simulink model "IEEE24bus_simplified"  (R2019b)
settings: Solver=ode23tb  StartTime=0.0  StopTime=100  MaxStep=1/60  RelTol=1e-4  AbsTol=1e-3  EnableMultiTasking=on
PreLoadFcn:
  | RTS96_data
values from neighbouring files (symbols this model uses):
  Efmax = 5    [IEEE24_bus.m]    (also in IEEE24bus_simplified_benchmark.m)
  Efmin = -5    [IEEE24_bus.m]    (also in IEEE24bus_simplified_benchmark.m)
  EXc_sys = [     0.06  25  0.2    0.0505  0.5685   0 0   0.091  0.35 ... (first row only)    [IEEE24bus_simplified_benchmark.m]
  FH1 = 12    [IEEE24bus_simplified_benchmark.m]
  FI1 = .9    (= 0.9)    [IEEE24bus_simplified_benchmark.m]
  FL1 = .1    (= 0.1)    [IEEE24bus_simplified_benchmark.m]
  KH1 = 100    [IEEE24bus_simplified_benchmark.m]
  KI1 = 1    [IEEE24_bus.m]    (also in IEEE24bus_simplified_benchmark.m = 20)
  KL1 = 10    [IEEE24bus_simplified_benchmark.m]
undefined symbols (not defined in the file or in its folder): D1, Delta
libraries: powerlib x157, sps_avr x11, powerlib_extras x1
(part 3 of 3)

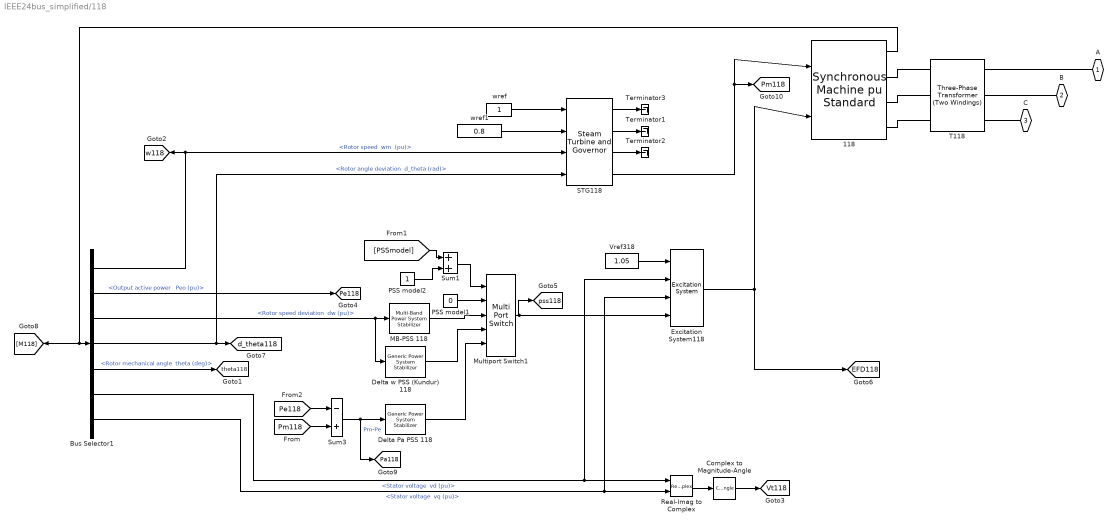
== system IEEE24bus_simplified/118 ==
  118 : powerlib/Machines/Synchronous Machine pu Standard  PresetModel=No  MechanicalLoad=Mechanical power Pm  ShowDetailedParameters=on  RotorType=Round  Units=per unit standard parameters  MeasurementBus=off  NominalParameters="[ 500E6  18e3   60]"  Reactances1="[ 1.782, 0.444, 0.283, 1.739, 1.201, 0.277,  0.275 ]"  Reactances2="[ 1.782, 0.444, 0.283, 1.739,  0.277,  0.275 ]"  dAxisTimeConstants=Open-circuit  qAxisTimeConstants=Open-circuit  TimeConstants1="[  6.070  0.055  0.035  ]"  TimeConstants2="[  6.070  0.055  1.5    0.152  ]"  TimeConstants3="[  6.070  0.055  0.035  ]"  TimeConstants4=[ 8.0, 0.03, 0.3371, 0.0295 ]  TimeConstants5=[ 1.01, 0.053, 0.1 ]  TimeConstants6=[ 1.3201, 0.023, 1.0, 0.07 ]  TimeConstants7="[  1.01  0.053  0.051266  ]"  TimeConstants8=[ 1.3201, 0.0231, 0.3371, 0.0295 ]  StatorResistance=0.0041  Mechanical="[ 1990/(500) 0  4 ]"  PolePairs=4  InitialConditions=[0 -39.3029 0.797786 0.797786 0.797786 -8.667 -128.667 111.333 2.00378]  SetSaturation=off  Saturation=[0.6404,0.7127,0.8441,0.9214,0.9956,1.082,1.19,1.316,1.457;0.7,0.7698,0.8872,0.9466,0.9969,1.046,1.1,1.151,1.201]  LoadFlowParameters=[1 400000000 18900 0 0]  TsPowergui=0  TsBlock=-1  IterativeModel=Forward Euler  IterativeDiscreteModel=Trapezoidal non iterative  BusType=PV  Pref=400E6  Qref=0  Qmin=-50e6  Qmax=200E6  PLF=0  QLF=0
      settings: SourceProductName=Simscape Electrical
  Bus Selector1 : BusSelector  OutputSignals="Mechanical.Rotor speed  wm  (pu),Output active power   Peo (pu),Mechanical.Rotor speed deviation  dw (pu),Mechanical.Rotor angle deviation  d_theta (rad),Mechanical.Rotor mechanical angle  theta (deg),dq0 components.Stator voltage  vd (pu),dq0 components.Stator voltage  vq (pu)"
  Complex to Magnitude-Angle : ComplexToMagnitudeAngle  Output=Magnitude
  Delta Pa PSS 118 : powerlib/Machines/Generic Power System Stabilizer  Tsensor=15e-3  K=2.5*1.25  Twashout=1  Tleadlag1=[60e-3 1]  Tleadlag2=[0 0]  VSlimits=[-0.15 0.15]  Vinit=0  Plot_On=off  MagdB_On=on  FreqRange=logspace(-2,2,500)
      settings: SourceProductName=Simscape Electrical  SourceProductBaseCode=PS
  Delta w PSS (Kundur) 118 : powerlib/Machines/Generic Power System Stabilizer  Tsensor=15e-3  K=30  Twashout=10  Tleadlag1=[50e-3 20e-3]  Tleadlag2=[3 5.4]  VSlimits=[-0.15 0.15]  Vinit=0  Plot_On=off  MagdB_On=on  FreqRange=logspace(-2,2,500)
      settings: SourceProductName=Simscape Electrical  SourceProductBaseCode=PS
  Excitation System118 : sps_avr/Excitation System  tr=EXc_sys(8,1)  reg="[ EXc_sys(8,2)   EXc_sys(8,3) ]"  exc="[ EXc_sys(8,4)  EXc_sys(8,5)]"  tgr="[ EXc_sys(8,6)  EXc_sys(8,7) ]"  damp="[ EXc_sys(8,8)   EXc_sys(8,9)]"  sat=[ 0, 0 ]  lim="[ Efmin Efmax   0 ]"  v0=[1.05,2.00378]
      settings: SourceProductName=Simscape Electrical  SourceProductBaseCode=PS
  MB-PSS 118 : powerlib/Machines/Multi-Band Power System Stabilizer  OperationMode=Simplified settings  Kg=G1  GL=[FL1 KL1]  GI=[FI1 KI1]  GH=[FH1 KH1]  GLd=[66 66 9.4]  TcLF=[1.667 2 0 0 0 0 2 2.4 0 0 0 0 1 1]  GId=[66 66 47.6]  TcIF=[1 1 0.25 0.3 0 0 1 1 0.3 0.36 0 0 0 0]  GHd=[66 66 233]  TcHF="[0.01 0.012 0 0 0 0  0.012 0.0144 0 0 0 0 1 1]"  LIM=[.075 .15 .15 .15]  Plot_On=off  MagdB_On=off  FreqRange=logspace(-2,2,500)
      settings: SourceProductName=Simscape Electrical  SourceProductBaseCode=PS
  Multiport Switch1 : MultiPortSwitch  Inputs=4  InputSameDT=on
  PSS model1 : Constant  Value=0
  PSS model2 : Constant
  Real-Imag to Complex : RealImagToComplex
  STG118 : powerlib/Machines/Steam Turbine and Governor  gentype=Tandem-compound (single mass)  reg1="[ 1  0.05    0 ]"  reg2="[ 0.001  0.15 ]"  reg3="[ -0.1  0.1  0  4.496 ]"  N=3600  turb1="[ 0  10   3.3   0.5   ]"  turb2="[   0   0.36    0.36   0.28   ]"  HA="[ 0.046  1.430  1.465   0.192 ]"  KA="[ 90.44  53.88  64.59   62.94  ]"  DA="[ 0.0115  0.3575  0.3663   0.0137  ]"  ini1=0.802609  ini2=[0.779316,-31.4247]
      settings: SourceProductName=Simscape Electrical  SourceProductBaseCode=PS
  Sum1 : Sum  SaturateOnIntegerOverflow=on  InputSameDT=on  OutDataTypeStr=Inherit: Same as first input
  Sum3 : Sum  Inputs=-+  SaturateOnIntegerOverflow=on  InputSameDT=on  OutDataTypeStr=Inherit: Same as first input
  T118 : powerlib/Elements/Three-Phase Transformer (Two Windings)  Winding1Connection=Delta (D1)  Winding2Connection=Yg  CoreType=Three single-phase transformers  SetSaturation=off  Hysteresis=off  DataFile='hysteresis'  SetInitialFlux=off  Measurements=None  UNITS=pu  NominalPower=[ 471E6 , 60 ]  Winding1=[ 18e3 , 1e-6 , 0 ]  Winding2=[ 230e3 , 0, 0.15 ]  Rm=500  Lm=500  L0=0.5  Saturation=[ 0,0 ; 0.0024,1.2 ; 1.0,1.52 ]  InitialFluxes=[ 0.8 , -0.8 , 0.7 ]  BreakLoop=off  DiscreteSolver=Trapezoidal iterative  DataType=off  TransfoNumber=0
      settings: SourceProductName=Simscape Electrical
  Terminator1 : Terminator
  Terminator2 : Terminator
  Terminator3 : Terminator
  Vref318 : Constant  Value=1.05
  wref : Constant
  wref1 : Constant  Value=0.8
  A : PMIOPort  Side=Right
  B : PMIOPort  Port=2  Side=Right
  C : PMIOPort  Port=3  Side=Right
  tag scope: EFD118=global, Pa118=global, Pe118=global, Pm118=global, Vt118=global, d_theta118=global, pss118=global, theta118=global, w118=global
  wires:
  Vref318/1 -> Excitation System118/1
  wref1/1 -> STG118/2
  wref/1 -> STG118/1
  118/1 -> [M118], Bus Selector1/1
  Bus Selector1/1 -> STG118/3, [w118]  "<Rotor speed  wm  (pu)>"
  Bus Selector1/2 -> [Pe118]  "<Output active power   Peo (pu)>"
  Bus Selector1/3 -> Delta w PSS (Kundur) 118/1, MB-PSS 118/1  "<Rotor speed deviation  dw (pu)>"
  Multiport Switch1/1 -> [pss118], Excitation System118/4
  PSS model2/1 -> Sum1/2
  Sum1/1 -> Multiport Switch1/1
  [PSSmodel] -> Sum1/1
  PSS model1/1 -> Multiport Switch1/2
  MB-PSS 118/1 -> Multiport Switch1/3
  Bus Selector1/4 -> [d_theta118], STG118/4  "<Rotor angle deviation  d_theta (rad)>"
  Bus Selector1/5 -> [theta118]  "<Rotor mechanical angle  theta (deg)>"
  Real-Imag to Complex/1 -> Complex to Magnitude-Angle/1
  Complex to Magnitude-Angle/1 -> [Vt118]
  Bus Selector1/6 -> Excitation System118/2, Real-Imag to Complex/1  "<Stator voltage  vd (pu)>"
  Bus Selector1/7 -> Excitation System118/3, Real-Imag to Complex/2  "<Stator voltage  vq (pu)>"
  Excitation System118/1 -> 118/2, [EFD118]
  STG118/1 -> Terminator3/1
  STG118/2 -> Terminator1/1
  STG118/3 -> Terminator2/1
  Sum3/1 -> [Pa118], Delta Pa PSS 118/1  "Pm-Pe"
  Delta Pa PSS 118/1 -> Multiport Switch1/5
  Delta w PSS (Kundur) 118/1 -> Multiport Switch1/4
  STG118/4 -> 118/1, [Pm118]
  [Pm118] -> Sum3/2
  [Pe118] -> Sum3/1
  connections:
  118/RConn3 -- T118/LConn3
  B/RConn1 -- T118/RConn2
  118/RConn2 -- T118/LConn2
  118/RConn1 -- T118/LConn1
  A/RConn1 -- T118/RConn1
  C/RConn1 -- T118/RConn3

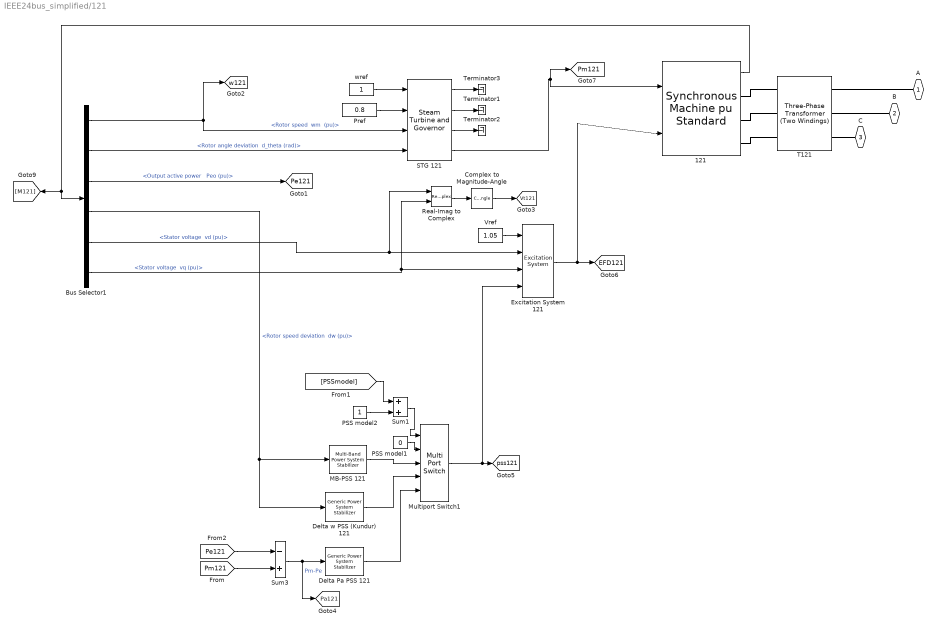
== system IEEE24bus_simplified/121 ==
  121 : powerlib/Machines/Synchronous Machine pu Standard  PresetModel=No  MechanicalLoad=Mechanical power Pm  ShowDetailedParameters=on  RotorType=Round  Units=per unit standard parameters  MeasurementBus=off  NominalParameters="[ 500E6  18e3   60]"  Reactances1="[ 1.782, 0.444, 0.283, 1.739, 1.201, 0.277,  0.275 ]"  Reactances2="[ 1.782, 0.444, 0.283, 1.739,  0.277,  0.275 ]"  dAxisTimeConstants=Open-circuit  qAxisTimeConstants=Open-circuit  TimeConstants1="[  6.070  0.055  0.035  ]"  TimeConstants2="[  6.070  0.055  1.5    0.152  ]"  TimeConstants3="[  6.070  0.055  0.035  ]"  TimeConstants4=[ 8.0, 0.03, 0.3371, 0.0295 ]  TimeConstants5=[ 1.01, 0.053, 0.1 ]  TimeConstants6=[ 1.3201, 0.023, 1.0, 0.07 ]  TimeConstants7="[  1.01  0.053  0.051266  ]"  TimeConstants8=[ 1.3201, 0.0231, 0.3371, 0.0295 ]  StatorResistance=0.0041  Mechanical="[ 1990/(500) 0  4 ]"  PolePairs=4  InitialConditions=[0 -38.0053 0.791351 0.791351 0.791351 -6.58132 -126.581 113.419 1.97426]  SetSaturation=off  Saturation=[0.6404,0.7127,0.8441,0.9214,0.9956,1.082,1.19,1.316,1.457;0.7,0.7698,0.8872,0.9466,0.9969,1.046,1.1,1.151,1.201]  LoadFlowParameters=[1 400000000 18900 0 0]  TsPowergui=0  TsBlock=-1  IterativeModel=Forward Euler  IterativeDiscreteModel=Trapezoidal non iterative  BusType=PV  Pref=400E6  Qref=0  Qmin=-50E6  Qmax=200E6  PLF=0  QLF=0
      settings: SourceProductName=Simscape Electrical
  Bus Selector1 : BusSelector  OutputSignals="Mechanical.Rotor speed  wm  (pu),Mechanical.Rotor angle deviation  d_theta (rad),Output active power   Peo (pu),Mechanical.Rotor speed deviation  dw (pu),dq0 components.Stator voltage  vd (pu),dq0 components.Stator voltage  vq (pu)"
  Complex to Magnitude-Angle : ComplexToMagnitudeAngle  Output=Magnitude
  Delta Pa PSS 121 : powerlib/Machines/Generic Power System Stabilizer  Tsensor=15e-3  K=2.5*1.25  Twashout=1  Tleadlag1=[60e-3 1]  Tleadlag2=[0 0]  VSlimits=[-0.15 0.15]  Vinit=0  Plot_On=off  MagdB_On=on  FreqRange=logspace(-2,2,500)
      settings: SourceProductName=Simscape Electrical  SourceProductBaseCode=PS
  Delta w PSS (Kundur) 121 : powerlib/Machines/Generic Power System Stabilizer  Tsensor=15e-3  K=30  Twashout=10  Tleadlag1=[50e-3 20e-3]  Tleadlag2=[3 5.4]  VSlimits=[-0.15 0.15]  Vinit=0  Plot_On=off  MagdB_On=on  FreqRange=logspace(-2,2,500)
      settings: SourceProductName=Simscape Electrical  SourceProductBaseCode=PS
  Excitation System 121 : sps_avr/Excitation System  tr=EXc_sys(9,1)  reg="[ EXc_sys(9,2)   EXc_sys(9,3) ]"  exc="[ EXc_sys(9,4)  EXc_sys(9,5)]"  tgr="[ EXc_sys(9,6)  EXc_sys(9,7) ]"  damp="[ EXc_sys(9,8)   EXc_sys(9,9)]"  sat=[ 0, 0 ]  lim="[ Efmin Efmax   0 ]"  v0=[1.05,1.97426]
      settings: SourceProductName=Simscape Electrical  SourceProductBaseCode=PS
  MB-PSS 121 : powerlib/Machines/Multi-Band Power System Stabilizer  OperationMode=Simplified settings  Kg=G1  GL=[FL1 KL1]  GI=[FI1 KI1]  GH=[FH1 KH1]  GLd=[66 66 9.4]  TcLF=[1.667 2 0 0 0 0 2 2.4 0 0 0 0 1 1]  GId=[66 66 47.6]  TcIF=[1 1 0.25 0.3 0 0 1 1 0.3 0.36 0 0 0 0]  GHd=[66 66 233]  TcHF="[0.01 0.012 0 0 0 0  0.012 0.0144 0 0 0 0 1 1]"  LIM=[.075 .15 .15 .15]  Plot_On=off  MagdB_On=off  FreqRange=logspace(-2,2,500)
      settings: SourceProductName=Simscape Electrical  SourceProductBaseCode=PS
  Multiport Switch1 : MultiPortSwitch  Inputs=4  InputSameDT=on
  PSS model1 : Constant  Value=0
  PSS model2 : Constant
  Pref : Constant  Value=0.8
  Real-Imag to Complex : RealImagToComplex
  STG 121 : powerlib/Machines/Steam Turbine and Governor  gentype=Tandem-compound (single mass)  reg1="[ 1  0.05    0 ]"  reg2="[ 0.001  0.15 ]"  reg3="[ -0.1  0.1  0  4.496 ]"  N=3600  turb1="[ 0  10   3.3   0.5   ]"  turb2="[   0   0.36    0.36   0.28   ]"  HA="[ 0.046  1.430  1.465   0.192 ]"  KA="[ 90.44  53.88  64.59   62.94  ]"  DA="[ 0.0115  0.3575  0.3663   0.0137  ]"  ini1=0.802568  ini2=[0.779316,-31.4247]
      settings: SourceProductName=Simscape Electrical  SourceProductBaseCode=PS
  Sum1 : Sum  SaturateOnIntegerOverflow=on  InputSameDT=on  OutDataTypeStr=Inherit: Same as first input
  Sum3 : Sum  Inputs=-+  SaturateOnIntegerOverflow=on  InputSameDT=on  OutDataTypeStr=Inherit: Same as first input
  T121 : powerlib/Elements/Three-Phase Transformer (Two Windings)  Winding1Connection=Delta (D1)  Winding2Connection=Yg  CoreType=Three single-phase transformers  SetSaturation=off  Hysteresis=off  DataFile='hysteresis'  SetInitialFlux=off  Measurements=None  UNITS=pu  NominalPower="[ 471E6  , 60 ]"  Winding1=[ 18e3 , 1e-6 , 0 ]  Winding2=[ 230e3 , 0, 0.15 ]  Rm=500  Lm=500  L0=0.5  Saturation=[ 0,0 ; 0.0024,1.2 ; 1.0,1.52 ]  InitialFluxes=[ 0.8 , -0.8 , 0.7 ]  BreakLoop=off  DiscreteSolver=Trapezoidal iterative  DataType=off  TransfoNumber=0
      settings: SourceProductName=Simscape Electrical
  Terminator1 : Terminator
  Terminator2 : Terminator
  Terminator3 : Terminator
  Vref : Constant  Value=1.05
  wref : Constant
  A : PMIOPort  Side=Right
  B : PMIOPort  Port=2  Side=Right
  C : PMIOPort  Port=3  Side=Right
  tag scope: EFD121=global, Pa121=global, Pe121=global, Pm121=global, Vt121=global, pss121=global, w121=global
  wires:
  Excitation System 121/1 -> 121/2, [EFD121]
  Vref/1 -> Excitation System 121/1
  STG 121/2 -> Terminator1/1
  STG 121/3 -> Terminator2/1
  STG 121/1 -> Terminator3/1
  wref/1 -> STG 121/1
  Pref/1 -> STG 121/2
  121/1 -> [M121], Bus Selector1/1
  Bus Selector1/1 -> STG 121/3, [w121]  "<Rotor speed  wm  (pu)>"
  Bus Selector1/2 -> STG 121/4  "<Rotor angle deviation  d_theta (rad)>"
  PSS model2/1 -> Sum1/2
  Sum1/1 -> Multiport Switch1/1
  Multiport Switch1/1 -> Excitation System 121/4, [pss121]
  [PSSmodel] -> Sum1/1
  PSS model1/1 -> Multiport Switch1/2
  MB-PSS 121/1 -> Multiport Switch1/3
  Bus Selector1/5 -> Real-Imag to Complex/1, Excitation System 121/2  "<Stator voltage  vd (pu)>"
  Bus Selector1/6 -> Real-Imag to Complex/2, Excitation System 121/3  "<Stator voltage  vq (pu)>"
  Real-Imag to Complex/1 -> Complex to Magnitude-Angle/1
  Complex to Magnitude-Angle/1 -> [Vt121]
  Bus Selector1/3 -> [Pe121]  "<Output active power   Peo (pu)>"
  Bus Selector1/4 -> Delta w PSS (Kundur) 121/1, MB-PSS 121/1  "<Rotor speed deviation  dw (pu)>"
  Sum3/1 -> [Pa121], Delta Pa PSS 121/1  "Pm-Pe"
  Delta Pa PSS 121/1 -> Multiport Switch1/5
  Delta w PSS (Kundur) 121/1 -> Multiport Switch1/4
  STG 121/4 -> [Pm121], 121/1
  [Pm121] -> Sum3/2
  [Pe121] -> Sum3/1
  connections:
  121/RConn3 -- T121/LConn3
  T121/RConn1 -- A/RConn1
  121/RConn2 -- T121/LConn2
  121/RConn1 -- T121/LConn1
  T121/RConn2 -- B/RConn1
  T121/RConn3 -- C/RConn1

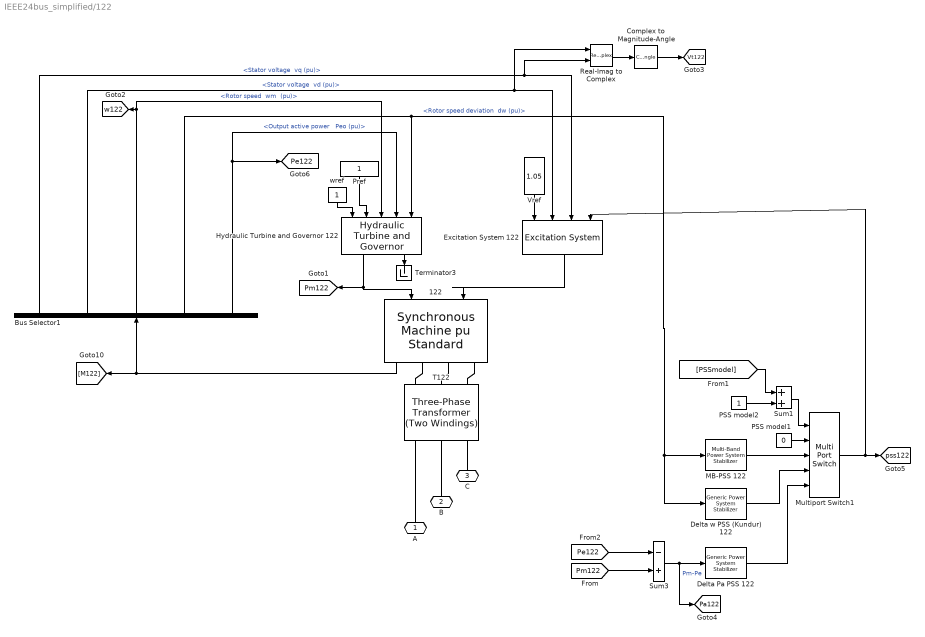
== system IEEE24bus_simplified/122 ==
  122 : powerlib/Machines/Synchronous Machine pu Standard  PresetModel=No  MechanicalLoad=Mechanical power Pm  ShowDetailedParameters=on  RotorType=Salient-pole  Units=per unit standard parameters  MeasurementBus=off  NominalParameters="[ 300E6  18e3   60]"  Reactances1="[ 0.995, 0.195, 0.155, 0.568,  0.568,  0.143,  0.160 ]"  Reactances2="[ 0.995, 0.195, 0.155, 0.568,  0.143,  0.160 ]"  dAxisTimeConstants=Open-circuit  qAxisTimeConstants=Open-circuit  TimeConstants1="[  9.2  0.03  0.06  ]"  TimeConstants2="[9.2     0.03    2       0.06]"  TimeConstants3="[  9.2  0.01  0.01  ]"  TimeConstants4="[  9.2  0.03  0.06  1 ]"  TimeConstants5=[ 1.01, 0.053, 0.1 ]  TimeConstants6=[ 1.3201, 0.023, 1.0, 0.07 ]  TimeConstants7="[  1.01  0.053  0.051266  ]"  TimeConstants8=[ 1.3201, 0.0231, 0.3371, 0.0295 ]  StatorResistance=0.0014  Mechanical="[ 1603/250 0  20]"  PolePairs=20  InitialConditions=[0 -51.0485 0.960961 0.960961 0.960961 5.59863 -114.401 125.599 1.47302]  SetSaturation=off  Saturation=[0.6404,0.7127,0.8441,0.9214,0.9956,1.082,1.19,1.316,1.457;0.7,0.7698,0.8872,0.9466,0.9969,1.046,1.1,1.151,1.201]  LoadFlowParameters=[1 300000000 18900 0 0]  TsPowergui=0  TsBlock=-1  IterativeModel=Forward Euler  IterativeDiscreteModel=Trapezoidal non iterative  BusType=PV  Pref=300E6  Qref=0  Qmin=-60E6  Qmax=96E6  PLF=0  QLF=0
      settings: SourceProductName=Simscape Electrical
  Bus Selector1 : BusSelector  OutputSignals="dq0 components.Stator voltage  vq (pu),dq0 components.Stator voltage  vd (pu),Mechanical.Rotor speed  wm  (pu),Mechanical.Rotor speed deviation  dw (pu),Output active power   Peo (pu)"
  Complex to Magnitude-Angle : ComplexToMagnitudeAngle  Output=Magnitude
  Delta Pa PSS 122 : powerlib/Machines/Generic Power System Stabilizer  Tsensor=15e-3  K=2.5*1.25  Twashout=1  Tleadlag1=[60e-3 1]  Tleadlag2=[0 0]  VSlimits=[-0.15 0.15]  Vinit=0  Plot_On=off  MagdB_On=on  FreqRange=logspace(-2,2,500)
      settings: SourceProductName=Simscape Electrical  SourceProductBaseCode=PS
  Delta w PSS (Kundur) 122 : powerlib/Machines/Generic Power System Stabilizer  Tsensor=15e-3  K=30  Twashout=10  Tleadlag1=[50e-3 20e-3]  Tleadlag2=[3 5.4]  VSlimits=[-0.15 0.15]  Vinit=0  Plot_On=off  MagdB_On=on  FreqRange=logspace(-2,2,500)
      settings: SourceProductName=Simscape Electrical  SourceProductBaseCode=PS
  Excitation System 122 : sps_avr/Excitation System  tr=EXc_sys(10,1)  reg="[ EXc_sys(10,2)   EXc_sys(10,3) ]"  exc="[ EXc_sys(10,4)  EXc_sys(10,5)]"  tgr="[ EXc_sys(10,6)  EXc_sys(10,7) ]"  damp="[ EXc_sys(10,8)   EXc_sys(10,9)]"  sat=[ 0, 0 ]  lim="[ Efmin Efmax   0 ]"  v0=[1.05,1.47302]
      settings: SourceProductName=Simscape Electrical  SourceProductBaseCode=PS
  Hydraulic Turbine and Governor 122 : powerlib/Machines/Hydraulic Turbine and Governor  sm="[ 10/3  0.07 ]"  gate="[  0.4  0.97518  -0.1  0.1 ]"  reg="[  0.05  1.163  0.105  0  0.01  ]"  hyd="[  0  2.67  ]"  dref=0  po=1.00129
      settings: SourceProductName=Simscape Electrical  SourceProductBaseCode=PS
  "MB-PSS 122 " : powerlib/Machines/Multi-Band Power System Stabilizer  OperationMode=Simplified settings  Kg=G1  GL=[FL1 KL1]  GI=[FI1 KI1]  GH=[FH1 KH1]  GLd=[66 66 9.4]  TcLF=[1.667 2 0 0 0 0 2 2.4 0 0 0 0 1 1]  GId=[66 66 47.6]  TcIF=[1 1 0.25 0.3 0 0 1 1 0.3 0.36 0 0 0 0]  GHd=[66 66 233]  TcHF="[0.01 0.012 0 0 0 0  0.012 0.0144 0 0 0 0 1 1]"  LIM=[.075 .15 .15 .15]  Plot_On=off  MagdB_On=off  FreqRange=logspace(-2,2,500)
      settings: SourceProductName=Simscape Electrical  SourceProductBaseCode=PS
  Multiport Switch1 : MultiPortSwitch  Inputs=4  InputSameDT=on
  PSS model1 : Constant  Value=0
  PSS model2 : Constant
  Pref : Constant
  Real-Imag to Complex : RealImagToComplex
  Sum1 : Sum  SaturateOnIntegerOverflow=on  InputSameDT=on  OutDataTypeStr=Inherit: Same as first input
  Sum3 : Sum  Inputs=-+  SaturateOnIntegerOverflow=on  InputSameDT=on  OutDataTypeStr=Inherit: Same as first input
  T122 : powerlib/Elements/Three-Phase Transformer (Two Windings)  Winding1Connection=Delta (D1)  Winding2Connection=Yg  CoreType=Three single-phase transformers  SetSaturation=off  Hysteresis=off  DataFile='hysteresis'  SetInitialFlux=off  Measurements=None  UNITS=pu  NominalPower=[ 318E6 , 60 ]  Winding1=[ 18e3 , 1e-6 , 0 ]  Winding2=[ 230e3 , 0, 0.1 ]  Rm=500  Lm=500  L0=0.5  Saturation=[ 0,0 ; 0.0024,1.2 ; 1.0,1.52 ]  InitialFluxes=[ 0.8 , -0.8 , 0.7 ]  BreakLoop=off  DiscreteSolver=Trapezoidal iterative  DataType=off  TransfoNumber=0
      settings: SourceProductName=Simscape Electrical
  Terminator3 : Terminator
  Vref : Constant  Value=1.05
  wref : Constant
  A : PMIOPort  Side=Right
  B : PMIOPort  Port=2  Side=Right
  C : PMIOPort  Port=3  Side=Right
  tag scope: Pa122=global, Pe122=global, Pm122=global, Vt122=global, pss122=global, w122=global
  wires:
  122/1 -> [M122], Bus Selector1/1
  Pref/1 -> Hydraulic Turbine and Governor 122/2
  wref/1 -> Hydraulic Turbine and Governor 122/1
  Vref/1 -> Excitation System 122/1
  Excitation System 122/1 -> 122/2
  PSS model2/1 -> Sum1/2
  Sum1/1 -> Multiport Switch1/1
  Multiport Switch1/1 -> Excitation System 122/4, [pss122]
  [PSSmodel] -> Sum1/1
  PSS model1/1 -> Multiport Switch1/2
  "MB-PSS 122 "/1 -> Multiport Switch1/3
  Bus Selector1/2 -> Real-Imag to Complex/1, Excitation System 122/2  "<Stator voltage  vd (pu)>"
  Bus Selector1/1 -> Real-Imag to Complex/2, Excitation System 122/3  "<Stator voltage  vq (pu)>"
  Real-Imag to Complex/1 -> Complex to Magnitude-Angle/1
  Complex to Magnitude-Angle/1 -> [Vt122]
  Bus Selector1/5 -> [Pe122], Hydraulic Turbine and Governor 122/4  "<Output active power   Peo (pu)>"
  Bus Selector1/4 -> Delta w PSS (Kundur) 122/1, "MB-PSS 122 "/1, Hydraulic Turbine and Governor 122/5  "<Rotor speed deviation  dw (pu)>"
  Sum3/1 -> [Pa122], Delta Pa PSS 122/1  "Pm-Pe"
  Delta Pa PSS 122/1 -> Multiport Switch1/5
  Delta w PSS (Kundur) 122/1 -> Multiport Switch1/4
  Hydraulic Turbine and Governor 122/1 -> 122/1, [Pm122]
  Bus Selector1/3 -> [w122], Hydraulic Turbine and Governor 122/3  "<Rotor speed  wm  (pu)>"
  [Pm122] -> Sum3/2
  [Pe122] -> Sum3/1
  Hydraulic Turbine and Governor 122/2 -> Terminator3/1
  connections:
  122/RConn3 -- T122/LConn3
  122/RConn1 -- T122/LConn1
  A/RConn1 -- T122/RConn1
  C/RConn1 -- T122/RConn3
  B/RConn1 -- T122/RConn2
  122/RConn2 -- T122/LConn2

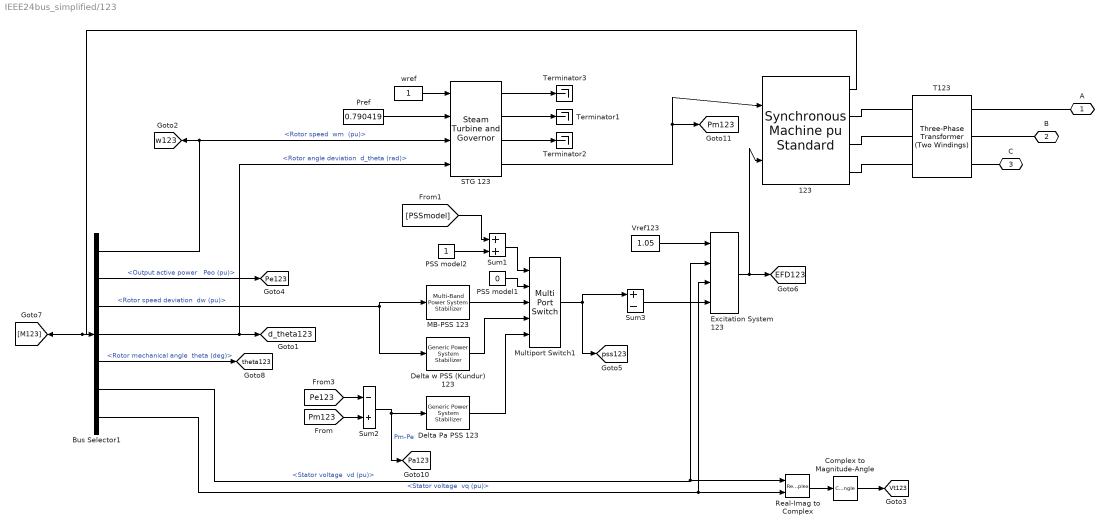
== system IEEE24bus_simplified/123 ==
  123 : powerlib/Machines/Synchronous Machine pu Standard  PresetModel=No  MechanicalLoad=Mechanical power Pm  ShowDetailedParameters=on  RotorType=Round  Units=per unit standard parameters  MeasurementBus=off  NominalParameters="[ 505E6  20e3   60]"  Reactances1="[ 2.183, 0.413, 0.339, 2.157, 1.285, 0.332,  0.246 ]"  Reactances2="[ 2.157, 1.285, 0.332, 2.157,  0.332,  0.246 ]"  dAxisTimeConstants=Open-circuit  qAxisTimeConstants=Open-circuit  TimeConstants1="[  5.690  0.041  0.144  ]"  TimeConstants2="[  5.690  0.041  1.5  0.144  ]"  TimeConstants3="[  5.690  0.041  0.144  ]"  TimeConstants4=[ 8.0, 0.03, 0.3371, 0.0295 ]  TimeConstants5=[ 1.01, 0.053, 0.1 ]  TimeConstants6=[ 1.3201, 0.023, 1.0, 0.07 ]  TimeConstants7="[  1.01  0.053  0.051266  ]"  TimeConstants8=[ 1.3201, 0.0231, 0.3371, 0.0295 ]  StatorResistance=0.0019  Mechanical="[ 2206.4/(835) 0  4 ]"  PolePairs=4  InitialConditions=[0 -36.4278 0.778296 0.778296 0.778296 -8.82761 -128.828 111.172 2.21318]  SetSaturation=off  Saturation=[0.6404,0.7127,0.8441,0.9214,0.9956,1.082,1.19,1.316,1.457;0.7,0.7698,0.8872,0.9466,0.9969,1.046,1.1,1.151,1.201]  LoadFlowParameters=[1 660000000 21000 0 0]  TsPowergui=0  TsBlock=-1  IterativeModel=Forward Euler  IterativeDiscreteModel=Trapezoidal non iterative  BusType=PV  Pref=660E6  Qref=0  Qmin=-195E6  Qmax=310E6  PLF=0  QLF=0
      settings: SourceProductName=Simscape Electrical
  Bus Selector1 : BusSelector  OutputSignals="Mechanical.Rotor speed  wm  (pu),Output active power   Peo (pu),Mechanical.Rotor speed deviation  dw (pu),Mechanical.Rotor angle deviation  d_theta (rad),Mechanical.Rotor mechanical angle  theta (deg),dq0 components.Stator voltage  vd (pu),dq0 components.Stator voltage  vq (pu)"
  Complex to Magnitude-Angle : ComplexToMagnitudeAngle  Output=Magnitude
  Delta Pa PSS 123 : powerlib/Machines/Generic Power System Stabilizer  Tsensor=15e-3  K=2.5*1.25  Twashout=1  Tleadlag1=[60e-3 1]  Tleadlag2=[0 0]  VSlimits=[-0.15 0.15]  Vinit=0  Plot_On=off  MagdB_On=on  FreqRange=logspace(-2,2,500)
      settings: SourceProductName=Simscape Electrical  SourceProductBaseCode=PS
  Delta w PSS (Kundur) 123 : powerlib/Machines/Generic Power System Stabilizer  Tsensor=15e-3  K=30  Twashout=10  Tleadlag1=[50e-3 20e-3]  Tleadlag2=[3 5.4]  VSlimits=[-0.15 0.15]  Vinit=0  Plot_On=off  MagdB_On=on  FreqRange=logspace(-2,2,500)
      settings: SourceProductName=Simscape Electrical  SourceProductBaseCode=PS
  Excitation System 123 : sps_avr/Excitation System  tr=EXc_sys(11,1)  reg="[ EXc_sys(11,2)   EXc_sys(11,3) ]"  exc="[ EXc_sys(11,4)  EXc_sys(11,5)]"  tgr="[ EXc_sys(11,6)  EXc_sys(11,7) ]"  damp="[ EXc_sys(11,8)   EXc_sys(11,9)]"  sat=[ 0, 0 ]  lim="[ Efmin Efmax   0 ]"  v0=[1.05,2.21318]
      settings: SourceProductName=Simscape Electrical  SourceProductBaseCode=PS
  MB-PSS 123 : powerlib/Machines/Multi-Band Power System Stabilizer  OperationMode=Simplified settings  Kg=G1  GL=[FL1 KL1]  GI=[FI1 KI1]  GH=[FH1 KH1]  GLd=[66 66 9.4]  TcLF=[1.667 2 0 0 0 0 2 2.4 0 0 0 0 1 1]  GId=[66 66 47.6]  TcIF=[1 1 0.25 0.3 0 0 1 1 0.3 0.36 0 0 0 0]  GHd=[66 66 233]  TcHF="[0.01 0.012 0 0 0 0  0.012 0.0144 0 0 0 0 1 1]"  LIM=[.075 .15 .15 .15]  Plot_On=off  MagdB_On=off  FreqRange=logspace(-2,2,500)
      settings: SourceProductName=Simscape Electrical  SourceProductBaseCode=PS
  Multiport Switch1 : MultiPortSwitch  Inputs=4  InputSameDT=on
  PSS model1 : Constant  Value=0
  PSS model2 : Constant
  Pref : Constant  Value=0.790419
  Real-Imag to Complex : RealImagToComplex
  STG 123 : powerlib/Machines/Steam Turbine and Governor  gentype=Tandem-compound (single mass)  reg1="[ 1  0.05    0 ]"  reg2="[ 0.001  0.15 ]"  reg3="[ -0.1  0.1  0  4.496 ]"  N=3600  turb1="[ 0  10   3.3   0.5   ]"  turb2="[   0   0.36    0.36   0.28   ]"  HA="[ 0.046  1.430  1.465   0.192 ]"  KA="[ 90.44  53.88  64.59   62.94  ]"  DA="[ 0.0115  0.3575  0.3663   0.0137  ]"  ini1=0.79157  ini2=[0.779316,-31.4247]
      settings: SourceProductName=Simscape Electrical  SourceProductBaseCode=PS
  Sum1 : Sum  SaturateOnIntegerOverflow=on  InputSameDT=on  OutDataTypeStr=Inherit: Same as first input
  Sum2 : Sum  Inputs=-+  SaturateOnIntegerOverflow=on  InputSameDT=on  OutDataTypeStr=Inherit: Same as first input
  Sum3 : Sum  Inputs=+-  SaturateOnIntegerOverflow=on  InputSameDT=on  OutDataTypeStr=Inherit: Same as first input
  T123 : powerlib/Elements/Three-Phase Transformer (Two Windings)  Winding1Connection=Yg  Winding2Connection=Delta (D1)  CoreType=Three single-phase transformers  SetSaturation=off  Hysteresis=off  DataFile='hysteresis'  SetInitialFlux=off  Measurements=None  UNITS=pu  NominalPower="[  776E6 , 60 ]"  Winding1=[ 230e3 , 0, 0.13 ]  Winding2=[ 20e3 , 1e-6 , 0 ]  Rm=500  Lm=500  L0=0.5  Saturation=[ 0,0 ; 0.0024,1.2 ; 1.0,1.52 ]  InitialFluxes=[ 0.8 , -0.8 , 0.7 ]  BreakLoop=off  DiscreteSolver=Trapezoidal iterative  DataType=off  TransfoNumber=0
      settings: SourceProductName=Simscape Electrical
  Terminator1 : Terminator
  Terminator2 : Terminator
  Terminator3 : Terminator
  Vref123 : Constant  Value=1.05
  wref : Constant
  A : PMIOPort  Side=Left
  B : PMIOPort  Port=2  Side=Left
  C : PMIOPort  Port=3  Side=Left
  tag scope: EFD123=global, Pa123=global, Pe123=global, Pm123=global, Vt123=global, d_theta123=global, pss123=global, theta123=global, w123=global
  wires:
  STG 123/4 -> [Pm123], 123/1
  123/1 -> [M123], Bus Selector1/1
  Vref123/1 -> Excitation System 123/1
  wref/1 -> STG 123/1
  Pref/1 -> STG 123/2
  Bus Selector1/1 -> STG 123/3, [w123]  "<Rotor speed  wm  (pu)>"
  Bus Selector1/2 -> [Pe123]  "<Output active power   Peo (pu)>"
  Excitation System 123/1 -> 123/2, [EFD123]
  Bus Selector1/4 -> [d_theta123], STG 123/4  "<Rotor angle deviation  d_theta (rad)>"
  Bus Selector1/5 -> [theta123]  "<Rotor mechanical angle  theta (deg)>"
  Multiport Switch1/1 -> Sum3/1, [pss123]
  Sum1/1 -> Multiport Switch1/1
  [PSSmodel] -> Sum1/1
  PSS model1/1 -> Multiport Switch1/2
  Sum3/1 -> Excitation System 123/4
  PSS model2/1 -> Sum1/2
  Bus Selector1/7 -> Real-Imag to Complex/2, Excitation System 123/3  "<Stator voltage  vq (pu)>"
  Bus Selector1/6 -> Excitation System 123/2, Real-Imag to Complex/1  "<Stator voltage  vd (pu)>"
  Real-Imag to Complex/1 -> Complex to Magnitude-Angle/1
  Complex to Magnitude-Angle/1 -> [Vt123]
  STG 123/1 -> Terminator3/1
  STG 123/2 -> Terminator1/1
  STG 123/3 -> Terminator2/1
  Bus Selector1/3 -> Delta w PSS (Kundur) 123/1, MB-PSS 123/1  "<Rotor speed deviation  dw (pu)>"
  Sum2/1 -> [Pa123], Delta Pa PSS 123/1  "Pm-Pe"
  Delta Pa PSS 123/1 -> Multiport Switch1/5
  Delta w PSS (Kundur) 123/1 -> Multiport Switch1/4
  [Pm123] -> Sum2/2
  [Pe123] -> Sum2/1
  MB-PSS 123/1 -> Multiport Switch1/3
  connections:
  123/RConn3 -- T123/RConn3
  123/RConn2 -- T123/RConn2
  C/RConn1 -- T123/LConn3
  B/RConn1 -- T123/LConn2
  123/RConn1 -- T123/RConn1
  A/RConn1 -- T123/LConn1
